simulink model "q1_a1"  (R2020b)
settings: Solver=FixedStepAuto  StartTime=0.0  StopTime=12  FixedStep=0.01  RelTol=1e-3
libraries: mpclib x1
settings Model: Creator=ALI  LastModifiedBy=ALI
settings DataIOCC: ReturnWorkspaceOutputs=off

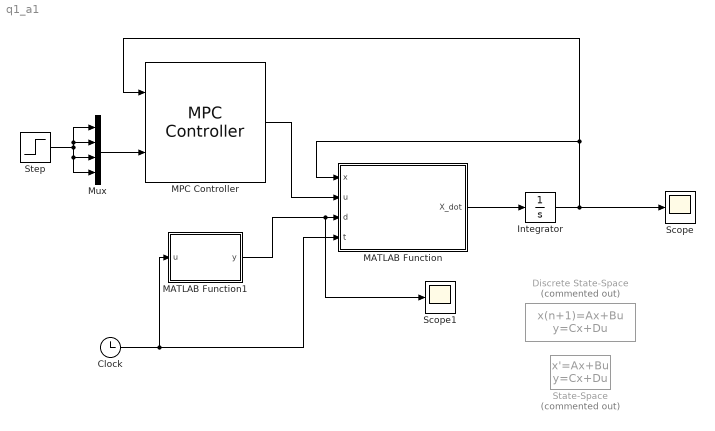
== system q1_a1 ==
  Clock : Clock
  Discrete State-Space : DiscreteStateSpace  Commented=on  SampleTime=-1
  Integrator : Integrator  InitialCondition=[0,0,0,0]
  MATLAB Function : MATLAB Function  TreatAsAtomicUnit=on
  MATLAB Function1 : MATLAB Function  TreatAsAtomicUnit=on
  MPC Controller : mpclib/MPC Controller  SCDEnableBlockLinearizationSpecification=on  mpcobj=mpc1  is_multiple=0  enable_value=0  return_u0=off  updateMPCinCallerWorkspace=on  md_inport=off  mv_inport=off  uref_inport=off  return_cost=off  return_mvseq=off  return_qpstatus=off  return_xseq=off  return_state=off  return_ovseq=off  state_inport=off  umin_inport=off  umax_inport=off  ymin_inport=off  ymax_inport=off  cc_inport=off  ywt_inport=off  uwt_inport=off  duwt_inport=off  rhoeps_inport=off  pm_inport=off  MaximumP=10  HorizonChoice=FixedHorizon  n_ts=0.01  n_p=100  n_mv=1  n_md=0  n_ud=0  n_mo=4  n_uo=0  BlockDataType=double  SampleTimeInherited=off  switch_inport=off
  Mux : Mux
  Scope : Scope
  Scope1 : Scope
  State-Space : StateSpace  Commented=on  InitialCondition=0
  Step : Step  SampleTime=0
  wires:
  MATLAB Function/1(X_dot) -> Integrator/1
  Integrator/1 -> MATLAB Function/1(x), MPC Controller/1, Scope/1
  Clock/1 -> MATLAB Function1/1(u), MATLAB Function/4(t)
  MATLAB Function1/1(y) -> Scope1/1, MATLAB Function/3(d)
  MPC Controller/1 -> MATLAB Function/2(u)
  Step/1 -> Mux/1, Mux/2, Mux/4, Mux/3
  Mux/1 -> MPC Controller/2

== matlab function q1_a1/MATLAB Function1 ==
  data: u input; y output
function y = distrubance(u)

if u>=4 & u<5
    y = (u-4);
elseif u>=5 & u<= 7
    y = 1;
elseif u>7 & u<8
    y = -u+8;
else
    y = 0;
end

== matlab function q1_a1/MATLAB Function ==
  data: x input; u input; X_dot output; d input; t input
function X_dot = state_space(x,u,d,t)

m_s = 2500;
m_u = 320;
k_s = 80000;
k_u = 500000;
c_s = 350;
c_u = 15020;


A = [
    0,          1,          0,          0;
    0,  -c_s/m_s,   -k_s/m_s,   c_s/m_s;
    0,          1,          0,         -1;
    -k_u/m_u, c_s/m_u,  (k_s+k_u)/m_u,  -(c_s+c_u)/m_u];

B1 = [0; c_s*c_u/(m_s*m_u); -c_u/m_u; c_u/m_u * (k_u/c_u - c_s/m_u - c_u/m_u)];
B2 = [0; 1/m_s; 0; -1/m_u];

X_dot = A*x + B1*d + B2*u;
